simulink model "fsco"  (Simulink 7.9)
settings: Solver=ode45  StartTime=0.0  StopTime=1000.0  RelTol=1e-3
libraries: simulink x2
settings Model: Creator=liang  LastModifiedBy=liang

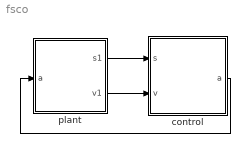
== system fsco ==
  control : Stateflow chart  TreatAsAtomicUnit=on
  plant : Subsystem
  wires:
  plant/1(s1) -> control/1(s)
  plant/2(v1) -> control/2(v)
  control/1(a) -> plant/1(a)

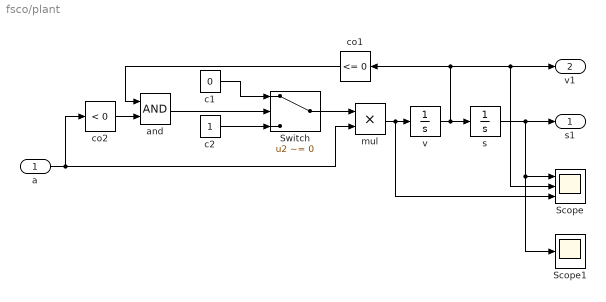
== system fsco/plant ==
  a : Inport
  Scope : Scope  NumInputPorts=3
      settings: YMin=-5~-5~-5  YMax=70000~260~5  MaxDataPoints=10000
  Scope1 : Scope
      settings: YMax=70000  MaxDataPoints=10000
  Switch : Switch  Criteria=u2 ~= 0
  and : Logic  AllPortsSameDT=off  OutDataTypeStr=boolean
  c1 : Constant  Value=0
  c2 : Constant
  co1 : simulink/Logic and Bit Operations/Compare To Zero  relop=<=  OutDataTypeStr=uint8
  co2 : simulink/Logic and Bit Operations/Compare To Zero  relop=<  OutDataTypeStr=uint8
  mul : Product  RndMeth=Zero
  s : Integrator
  v : Integrator
  s1 : Outport
  v1 : Outport  Port=2
  wires:
  v/1 -> s/1, co1/1, v1/1, Scope/2
  s/1 -> s1/1, Scope/1, Scope1/1
  mul/1 -> v/1, Scope/3
  Switch/1 -> mul/1
  a/1 -> co2/1, mul/2
  co1/1 -> and/1
  co2/1 -> and/2
  c1/1 -> Switch/1
  and/1 -> Switch/2
  c2/1 -> Switch/3

== stateflow chart control ==
  settings: updateMethod=DISCRETE  sampleTime=0.125
  state Driver [parallel]
    settings: executionOrder=4
    Driver -> Driver : CONFR/CONF
  state TCC [parallel]
    settings: executionOrder=3
    TCC -> TCC : MAA2/MAA2c
  state RBC [parallel]
    settings: executionOrder=2
    RBC -> RBC [order 2] : MAA3/MAA3c
    RBC -> RBC [order 1] : LUA/LU
  state Train [parallel]
    settings: executionOrder=1
    state l2
      l2 -> (junction 17) [order 3] : MAA2c{FMA2();FB2()}
      (junction 17) -> l2 [order 1] : [fv>=vr1]/a=C_b
      (junction 17) -> l2 [order 2] : [fv>=vr2]/a=C_a
      l2 -> (junction 17) [order 2] : [i==0 & s>200]/i=1;FB2();LUA
      l2 -> (junction 17) [order 4] : [s>e22]/mode2=mode23;FB2();MAA2
      l2 -> (junction 17) [order 5] : {FB2()}
      (junction 17) -> l2 [order 3] : /a=C_A
      l2 -> (junction 17) [order 1] : LU/i=2;FB2()
    state l2a
      (junction 16) -> l2a [order 3] : /a=C_A
      l2a -> (junction 16) [order 4] : [s>e32]/mode3=mode33;FB22();MAA3
      (junction 16) -> l2a [order 2] : [fv>=vr2]/a=C_a
      l2a -> (junction 16) [order 1] : MAA3c{FMA3();FB22()}
      (junction 16) -> l2a [order 1] : [fv>=vr1]/a=C_b
      l2a -> (junction 16) [order 5] : {FB22()}
      l2a -> (junction 16) [order 3] : [s>e22]/mode2=mode23;FB22();MAA2
      l2a -> (junction 16) [order 2] : MAA2c{FMA2();FB22()}
    state l3
      l3 -> (junction 15) [order 1] : CONF{v321=45;v322=40;FB3()}
      l3 -> (junction 15) [order 5] : {FB3()}
      (junction 15) -> l3 [order 1] : [fv>=vr1]/a=C_b
      l3 -> (junction 15) [order 4] : [s>e32]/mode3=mode33;MAA3
      l3 -> (junction 15) [order 3] : MAA3c{FMA3();FB3()}
      (junction 15) -> l3 [order 2] : [fv>=vr2]/a=C_a
      (junction 15) -> l3 [order 3] : /a=C_A
      l3 -> (junction 15) [order 2] : [mode32==1 & v321==0]/FB3();CONFR
    l2 -> l2a [order 1] : [i==2 & s>=x1]/a=C_b
    (default) -> l2
    l2a -> l3 [order 1] : [s>x2]
  data: vr2 local double; vr1 local double; v332 local double =0; v331 local double =0; v322 local double =250; v321 local double =255; v312 local double =250; v311 local double =255; v232 local double =40; v231 local double =45; v222 local double =100; v221 local double =105; v212 local double =100; v211 local double =105; e33 local double =96000; e32 local double =64000; e31 local double =32000; e23 local double =96000; e22 local double =64000; e21 local double =32000; mode33 local double =1; mode32 local double =0; mode31 local double =0; mode23 local double =1; mode22 local double =0; mode21 local double =0; mode3 local double =0; mode2 local double =0; C_b constant double =-1; C_A constant double =1; C_a constant double =-0.2; i local double =2; fv local double; x2 local double =64000; x1 local double =32000; T local double; s input double; v input double; a output double =0
  events: CONFR local EITHER_EDGE_EVENT; MAA2 local EITHER_EDGE_EVENT; MAA2c local EITHER_EDGE_EVENT; MAA3 local EITHER_EDGE_EVENT; MAA3c local EITHER_EDGE_EVENT; LU local EITHER_EDGE_EVENT; LUA local EITHER_EDGE_EVENT; CONF local EITHER_EDGE_EVENT
  function FMA2:
    | function FMA2()
    | 
    | e21 = e22;
    | e22 = e23;
    | e23 = (e23 + 32000);
    | v211 = v221;
    | v212 = v222;
    | v221 = v231;
    | v222 = v232;
    | v231 = 105;
    | v232 = 100;
    | mode21 = mode22;
    | mode22 = mode23;
    | mode23 = 0;
  function FB22:
    | function FB22()
    | T = 1/8;
    | 
    | vr1 = ((v211 + 2*T) * (v211 + 2*T));
    | vr1 = min(vr1, (v311 + 2*T) * (v311 + 2*T));
    | vr1 = min(vr1, ((2*C_b*s-2*C_b*e33) + 2*T*T));
    | vr1 = min(vr1, ((v331*v331-2*C_b*e32)+2*C_b*s + 2*T*T));
    | 
    | vr2 = ((v212 + 2*T) * (v212 + 2*T));
    | vr2 = min(vr2,(v312 + 2*T) * (v312 + 2*T));
    | vr2 = min(vr2, ((v332 *v332-2*C_b*e32)+2*C_b*s + 2*T*T));
    | vr2 = min(vr2, ((2*C_b*s-2*C_b*e33) + 2*T*T));
    | 
    | fv = (v*v + 1/2*v + 4*T*T);
  function FB2:
    | function FB2
    | T = 1/8;
    | 
    | vr1 = ((v211 + 2*T) * (v211 + 2*T));
    | vr1 = min(vr1, ((v221*v221-2*C_b*e21)+2*C_b*s + 2*T*T));
    | vr1 = min(vr1, ((v231*v231-2*C_b*e22)+2*C_b*s + 2*T*T));
    | vr1 = min(vr1, ((2*C_b*s-2*C_b*e32) + 2*T*T));
    | 
    | vr2 = ((v212 + 2*T) * (v212 + 2*T));
    | vr2 = min(vr2, ((v222 *v222-2*C_b*e21)+2*C_b*s + 2*T*T));
    | vr2 = min(vr2, ((v232 *v232-2*C_b*e22)+2*C_b*s + 2*T*T));
    | vr2 = min(vr2, ((2*C_b*s-2*C_b*e23) + 2*T*T));
    | 
    | fv = (v*v + 1/2*v + 4*T*T);
  function FMA3:
    | function FMA3
    | 
    | e31 = e32;
    | e32 = e33;
    | e33 = (e33 + 32000);
    | v311 = v321;
    | v312 = v322;
    | v321 = v331;
    | v322 = v332;
    | v331 = 255;
    | v332 = 250;
    | mode31 = mode32;
    | mode32 = mode33;
    | mode33 = 0;
  function FB3:
    | function FB3
    | T = 1/8;
    | 
    | vr1 = ((v311 + 2*T) * (v311 + 2*T));
    | vr1 = min(vr1, ((v321*v321-2*C_b*e31)+2*C_b*s + 2*T*T));
    | vr1 = min(vr1, ((v331*v331-2*C_b*e32)+2*C_b*s + 2*T*T));
    | vr1 = min(vr1, ((2*C_b*s-2*C_b*e33) + 2*T*T));
    | 
    | vr2 = ((v312 + 2*T) * (v312 + 2*T));
    | vr2 = min(vr2, ((v322 *v322-2*C_b*e31)+2*C_b*s + 2*T*T));
    | vr2 = min(vr2, ((v332 *v332-2*C_b*e32)+2*C_b*s + 2*T*T));
    | vr2 = min(vr2, ((2*C_b*s-2*C_b*e33) + 2*T*T));
    | 
    | fv=((v + 2*T)*(v + 2*T));
